simulink model "CAMFC2_04_simple_Formation"  (R2018b)
settings: Solver=ode23  StartTime=0.0  StopTime=20  RelTol=1e-3  EnableMultiTasking=on
InitFcn:
  | constant_CAMFC2_04_Simple_Formation
values from neighbouring files (symbols this model uses):
  alpha = 0.1    [constant_CAMFC2_01_WMR01.m]    (also in constant_CAMFC2_04_Comp.m = 0.01; constant_CAMFC2_04_Quad_03.m; constant_CAMFC2_04_Simple.m = 0.01; constant_CAMFC2_04_Simple_DoubleIntegrator.m = 0.01)
  AN = [     0 1 0 0 ... (first row only)    [constant_CAMFC2_01_WMR01.m]    (also in constant_CAMFC2_04_Comp.m = [     0 1 0 0 1; constant_CAMFC2_04_Quad_03.m; constant_CAMFC2_04_Simple.m; constant_CAMFC2_04_Simple_DoubleIntegrator.m)
  BN = [     1 0 0 0 ... (first row only)    [constant_CAMFC2_01_WMR01.m]    (also in constant_CAMFC2_04_Comp.m = [     0 0 0 0 0; constant_CAMFC2_04_Quad_03.m; constant_CAMFC2_04_Simple.m; constant_CAMFC2_04_Simple_DoubleIntegrator.m)
  chi = [0 0 0 0 ... (first row only)    [constant_CAMFC2_01_WMR01.m]    (also in constant_CAMFC2_04_Comp.m = X_m*ones(n0,1); constant_CAMFC2_04_Quad_03.m = X_m*ones(n0,1); constant_CAMFC2_04_Simple.m = X_m*ones(n0,1); constant_CAMFC2_04_Simple_DoubleIntegrator.m = X_m*ones(n0,1))
  epsilon_struct = struct('data',epsilon_InitVal)    [constant_CAMFC2_01_WMR01.m]    (also in constant_CAMFC2_04_Comp.m; constant_CAMFC2_04_Quad_03.m; constant_CAMFC2_04_Simple.m; constant_CAMFC2_04_Simple_DoubleIntegrator.m)
  gama1 = 1e4*diag([1e-6*ones(2,1);1e0*ones(2,1)])    [constant_CAMFC2_01_WMR01.m]    (also in constant_CAMFC2_04_Comp.m = 1e+3*diag([1e-6;1e-0]); constant_CAMFC2_04_Quad_03.m = 1e+2*diag(1e-0*ones(n0,1)); constant_CAMFC2_04_Simple.m = 1e+2*diag([1e-0;1e-0]); constant_CAMFC2_04_Simple_Formation.m = 1e+2*diag([1e-0;1e-0]))
  gama2 = 1e-2*diag([1e-6*ones(2,1);1e0*ones(2,1)])    [constant_CAMFC2_01_WMR01.m]    (also in constant_CAMFC2_04_Comp.m = 1e+0*diag([1e-6;1e-0]); constant_CAMFC2_04_Quad_03.m = 1e+0*diag(1e-0*ones(n0,1)); constant_CAMFC2_04_Simple.m = 1e+1*diag([1e-0;1e-0]); constant_CAMFC2_04_Simple_Formation.m = 1e+1*diag([1e-0;1e-0]))
  H = L + BN    [constant_CAMFC2_01_WMR01.m]    (also in constant_CAMFC2_04_Comp.m; constant_CAMFC2_04_Quad_03.m; constant_CAMFC2_04_Simple.m; constant_CAMFC2_04_Simple_DoubleIntegrator.m)
  k1 = 1    [constant_CAMFC2_01_WMR01.m]    (also in constant_CAMFC2_04_Comp.m; constant_CAMFC2_04_Quad_03.m = 50; constant_CAMFC2_04_Simple.m; constant_CAMFC2_04_Simple_DoubleIntegrator.m)
  k2 = 1    [constant_CAMFC2_01_WMR01.m]    (also in constant_CAMFC2_04_Comp.m; constant_CAMFC2_04_Quad_03.m; constant_CAMFC2_04_Simple.m; constant_CAMFC2_04_Simple_DoubleIntegrator.m)
  n = 4    [constant_CAMFC2_01_WMR01.m]    (also in constant_CAMFC2_04_Comp.m = 2; constant_CAMFC2_04_Quad_03.m = 6; constant_CAMFC2_04_Simple.m = 2; constant_CAMFC2_04_Simple_DoubleIntegrator.m = 2)
  N = 4    [constant_CAMFC2_01_WMR01.m]    (also in constant_CAMFC2_04_Comp.m = 5; constant_CAMFC2_04_Quad_03.m; constant_CAMFC2_04_Simple.m; constant_CAMFC2_04_Simple_DoubleIntegrator.m)
  n0 = 2    [constant_CAMFC2_01_WMR01.m]    (also in constant_CAMFC2_04_Comp.m = 1; constant_CAMFC2_04_Quad_03.m = 3; constant_CAMFC2_04_Simple.m; constant_CAMFC2_04_Simple_DoubleIntegrator.m = 1)
  Observer_Gain = 100    [constant_CAMFC2_01_WMR01.m]    (also in constant_CAMFC2_04_Comp.m = 10; constant_CAMFC2_04_Quad_03.m = 1; constant_CAMFC2_04_Simple.m; constant_CAMFC2_04_Simple_DoubleIntegrator.m)
  Observer_Gain1 = 100    [constant_CAMFC2_01_WMR01.m]    (also in constant_CAMFC2_04_Comp.m = 10; constant_CAMFC2_04_Quad_03.m = 1; constant_CAMFC2_04_Simple.m; constant_CAMFC2_04_Simple_DoubleIntegrator.m)
  Omega = [0 0 ... (first row only)    [constant_CAMFC2_04_Comp.m]    (also in constant_CAMFC2_04_Simple.m; constant_CAMFC2_04_Simple_DoubleIntegrator.m; constant_CAMFC2_04_Simple_DoubleIntegrator_02.m; constant_CAMFC2_04_Simple_Formation.m)
  P_struct = struct('data',P_InitVal)    [constant_CAMFC2_01_WMR01.m]    (also in constant_CAMFC2_04_Comp.m; constant_CAMFC2_04_Quad_03.m; constant_CAMFC2_04_Simple.m; constant_CAMFC2_04_Simple_DoubleIntegrator.m)
  Q = 1e-0*eye(n)    [constant_CAMFC2_01_WMR01.m]    (also in constant_CAMFC2_04_Comp.m = 1.0e+2*eye(n); constant_CAMFC2_04_Quad_03.m = 1e-0*eye(n0); constant_CAMFC2_04_Simple.m = 1.0e+1*eye(n); constant_CAMFC2_04_Simple_Formation.m = 1.0e+1*eye(n))
  rho1 = 1e-1    (= 0.1)    [constant_CAMFC2_01_WMR01.m]    (also in constant_CAMFC2_04_Comp.m = 1; constant_CAMFC2_04_Quad_03.m = 1; constant_CAMFC2_04_Simple.m = 1; constant_CAMFC2_04_Simple_DoubleIntegrator.m = 1)
  rho2 = 1e-3    (= 0.001)    [constant_CAMFC2_01_WMR01.m]    (also in constant_CAMFC2_04_Comp.m = 1; constant_CAMFC2_04_Quad_03.m = 1; constant_CAMFC2_04_Simple.m = 1; constant_CAMFC2_04_Simple_DoubleIntegrator.m = 10)
  T_struct = struct('data',T_InitVal)    [constant_CAMFC2_01_WMR01.m]    (also in constant_CAMFC2_04_Comp.m; constant_CAMFC2_04_Quad_03.m; constant_CAMFC2_04_Simple.m; constant_CAMFC2_04_Simple_DoubleIntegrator.m)
  Upsilon_M = Upsilon_m*ones(n,1)    [constant_CAMFC2_01_WMR01.m]    (also in constant_CAMFC2_04_Comp.m; constant_CAMFC2_04_Quad_03.m = Upsilon_m*ones(n0,1); constant_CAMFC2_04_Simple.m; constant_CAMFC2_04_Simple_DoubleIntegrator.m)
(part 1 of 3)
settings Model: ExtModeTrigDuration=100  Creator=hp  LastModifiedBy=ali
settings DataIOCC: LimitDataPoints=on  SaveFinalState=on  SaveFormat=StructureWithTime  SaveOutput=off  SaveState=on  StateSaveName=tmp_raccel_xout  SignalLoggingName=tmp_raccel_logsout
settings OptimizationCC: EfficientMapNaN2IntZero=off  LifeSpan=inf
settings DebuggingCC: UnderspecifiedInitializationDetection=Classic  MergeDetectMultiDrivingBlocksExec=none  SFUnexpectedBacktrackingDiag=warning  SFNoUnconditionalDefaultTransitionDiag=warning  SFExecutionAtInitializationDiag=none
settings HardwareCC: ProdBitPerPointer=32  ProdBitPerSizeT=32  ProdBitPerPtrDiffT=32  ProdLargestAtomicFloat=None  ProdIntDivRoundTo=Undefined  ProdEndianess=Unspecified  ProdWordSize=32  ProdHWDeviceType=32-bit Generic  TargetBitPerPointer=64  TargetBitPerSizeT=64  TargetBitPerPtrDiffT=64  TargetLongLongMode=on  TargetIntDivRoundTo=Zero  TargetEndianess=LittleEndian  TargetWordSize=64  TargetHWDeviceType=MATLAB Host  ProdEqTarget=off
settings ModelReferenceCC: PropagateSignalLabelsOutOfModel=off
settings SFSimCC: SimUseLocalCustomCode=off
settings RTWCC: SystemTargetFile=raccel.tlc  TemplateMakefile=raccel_default_tmf  RTWVerbose=off  RTWUseLocalCustomCode=off  RTWUseSimCustomCode=on
settings CodeAppCC: GenerateComments=off  MaxIdLength=128  MangleLength=10  SimulinkBlockComments=off
settings RaccelTargetCC: GeneratePreprocessorConditionals=Use local settings  MultiInstanceERTCode=off  PreserveStateflowLocalDataDimensions=off  ExtModeMexArgs='', 0, 54523  ENABLE_SLEXEC_SSBRIDGE=0  RTWCAPIParams=on
settings ConfigComp: CovMetricSettings=dw  CovHtmlReporting=on  CovSaveCumulativeToWorkspaceVar=on  CovSaveSingleToWorkspaceVar=on  CovExternalEMLEnable=off

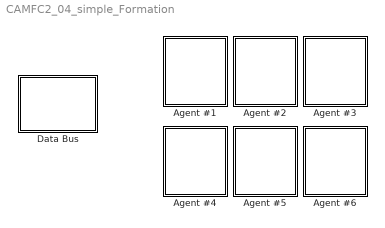
== system CAMFC2_04_simple_Formation ==
  Agent #1 : Subsystem
  Agent #2 : Subsystem
  Agent #3 : Subsystem
  Agent #4 : Subsystem
  Agent #5 : Subsystem
  Agent #6 : Subsystem
  "Data Bus " : Subsystem

== system CAMFC2_04_simple_Formation/Agent #1 ==
  Agent # : Constant
  Controller interpreter : MATLAB Function  TreatAsAtomicUnit=on
  Decenteralized Cooperaive Controller #1 : Subsystem
  Formation Plant : Subsystem
  tag scope: u1=global, x1=global
  wires:
  Decenteralized Cooperaive Controller #1/1(U1) -> Controller interpreter/1(U)
  Agent #/1 -> Decenteralized Cooperaive Controller #1/1(Agent #)
  Formation Plant/1(Y) -> [x1]
  Controller interpreter/1(u) -> Formation Plant/1(U), [u1]

== system CAMFC2_04_simple_Formation/Agent #2 ==
  Agent # : Constant  Value=2
  Controller interpreter : MATLAB Function  TreatAsAtomicUnit=on
  Decenteralized Cooperaive Controller #2 : Subsystem
  Formation Plant : Subsystem
  tag scope: u2=global, x2=global
  wires:
  Agent #/1 -> Decenteralized Cooperaive Controller #2/1(Agent #)
  Controller interpreter/1(u) -> Formation Plant/1(U), [u2]
  Formation Plant/1(Y) -> [x2]
  Decenteralized Cooperaive Controller #2/1(U2) -> Controller interpreter/1(U)

== system CAMFC2_04_simple_Formation/Agent #3 ==
  Agent # : Constant  Value=3
  Controller interpreter : MATLAB Function  TreatAsAtomicUnit=on
  Decenteralized Cooperaive Controller #3 : Subsystem
  Formation Plant : Subsystem
  tag scope: u3=global, x3=global
  wires:
  Agent #/1 -> Decenteralized Cooperaive Controller #3/1(Agent #)
  Formation Plant/1(Y) -> [x3]
  Decenteralized Cooperaive Controller #3/1(U3) -> Controller interpreter/1(U)
  Controller interpreter/1(u) -> Formation Plant/1(U), [u3]

== system CAMFC2_04_simple_Formation/Agent #4 ==
  Agent # : Constant  Value=4
  Controller interpreter : MATLAB Function  TreatAsAtomicUnit=on
  Decenteralized Cooperaive Controller #4 : Subsystem
  Formation Plant : Subsystem
  tag scope: u4=global, x4=global
  wires:
  Formation Plant/1(Y) -> [x4]
  Agent #/1 -> Decenteralized Cooperaive Controller #4/1(Agent #)
  Decenteralized Cooperaive Controller #4/1(U4) -> Controller interpreter/1(U)
  Controller interpreter/1(u) -> Formation Plant/1(U), [u4]

== system CAMFC2_04_simple_Formation/Agent #5 ==
  Agent # : Constant  Value=5
  Controller interpreter : MATLAB Function  TreatAsAtomicUnit=on
  Decenteralized Cooperaive Controller #5 : Subsystem
  Formation Plant : Subsystem
  tag scope: u5=global, x5=global
  wires:
  Controller interpreter/1(u) -> [u5], Formation Plant/1(U)
  Decenteralized Cooperaive Controller #5/1(U5) -> Controller interpreter/1(U)
  Agent #/1 -> Decenteralized Cooperaive Controller #5/1(Agent #)
  Formation Plant/1(Y) -> [x5]

== system CAMFC2_04_simple_Formation/Agent #6 ==
  Agent # : Constant  Value=6
  Controller interpreter : MATLAB Function  TreatAsAtomicUnit=on
  Decenteralized Cooperaive Controller #6 : Subsystem
  Formation Plant : Subsystem
  tag scope: u6=global, x6=global
  wires:
  Formation Plant/1(Y) -> [x6]
  Agent #/1 -> Decenteralized Cooperaive Controller #6/1(Agent #)
  Decenteralized Cooperaive Controller #6/1(U6) -> Controller interpreter/1(U)
  Controller interpreter/1(u) -> Formation Plant/1(U), [u6]

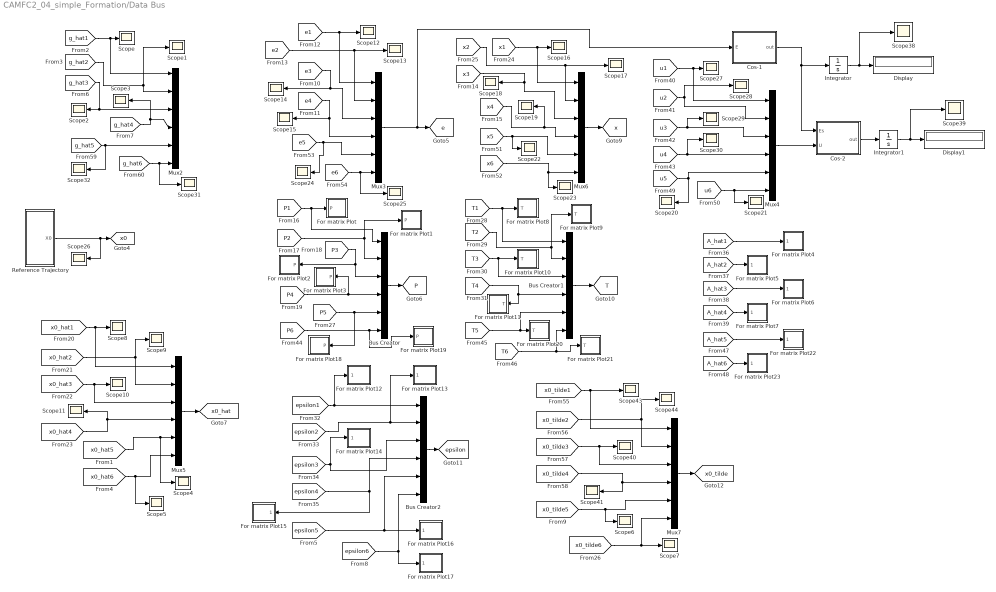
== system CAMFC2_04_simple_Formation/Data Bus  ==
  Bus Creator : BusCreator  Inputs=6  OutDataTypeStr=Bus: P_bus
  Bus Creator1 : BusCreator  Inputs=6  OutDataTypeStr=Bus: T_bus
  Bus Creator2 : BusCreator  Inputs=6  OutDataTypeStr=Bus: epsilon_bus
  Cos-1 : MATLAB Function  TreatAsAtomicUnit=on
  Cos-2 : MATLAB Function  TreatAsAtomicUnit=on
  Display : Display
  Display1 : Display
  For matrix Plot : Subsystem
  For matrix Plot1 : Subsystem
  For matrix Plot10 : Subsystem
  For matrix Plot11 : Subsystem
  For matrix Plot12 : Subsystem
  For matrix Plot13 : Subsystem
  For matrix Plot14 : Subsystem
  For matrix Plot15 : Subsystem
  For matrix Plot16 : Subsystem
  For matrix Plot17 : Subsystem
  For matrix Plot18 : Subsystem
  For matrix Plot19 : Subsystem
  For matrix Plot2 : Subsystem
  For matrix Plot20 : Subsystem
  For matrix Plot21 : Subsystem
  For matrix Plot22 : Subsystem
  For matrix Plot23 : Subsystem
  For matrix Plot3 : Subsystem
  For matrix Plot4 : Subsystem
  For matrix Plot5 : Subsystem
  For matrix Plot6 : Subsystem
  For matrix Plot7 : Subsystem
  For matrix Plot8 : Subsystem
  For matrix Plot9 : Subsystem
  Integrator : Integrator
  Integrator1 : Integrator
  Mux{2..7} (6 alike) : Mux  Inputs=6
  Reference Trajectory : Subsystem
  Scope{,1..32,38..41,43..44} (39 alike) : Scope
  tag scope: P=global, T=global, e=global, epsilon=global, x0=global, x0_hat=global, x0_tilde=global, x=global
  wires:
  [g_hat2] -> Scope1/1, Mux2/2
  [g_hat1] -> Mux2/1, Scope/1
  [e2] -> Mux3/2, Scope13/1
  [e1] -> Mux3/1, Scope12/1
  Mux3/1 -> Cos-1/1(E), [e]
  [P2] -> Bus Creator/2, For matrix Plot1/1(P)
  [P1] -> Bus Creator/1, For matrix Plot/1(P)
  Bus Creator/1 -> [P]
  [x0_hat2] -> Scope9/1, Mux5/2
  [x0_hat1] -> Mux5/1, Scope8/1
  Mux5/1 -> [x0_hat]
  Reference Trajectory/1(X0) -> [x0], Scope26/1
  [x2] -> Mux6/2, Scope17/1
  [x1] -> Mux6/1, Scope16/1
  Mux6/1 -> [x]
  [g_hat3] -> Mux2/3, Scope2/1
  [g_hat4] -> Mux2/4, Scope3/1
  [e3] -> Mux3/3, Scope14/1
  [e4] -> Mux3/4, Scope15/1
  [x3] -> Mux6/3, Scope18/1
  [x4] -> Mux6/4, Scope19/1
  [P3] -> Bus Creator/3, For matrix Plot2/1(P)
  [P4] -> For matrix Plot3/1(P), Bus Creator/4
  [x0_hat3] -> Mux5/3, Scope10/1
  [x0_hat4] -> Scope11/1, Mux5/4
  [T2] -> Bus Creator1/2, For matrix Plot9/1(T)
  [T1] -> Bus Creator1/1, For matrix Plot8/1(T)
  Bus Creator1/1 -> [T]
  [T3] -> Bus Creator1/3, For matrix Plot10/1(T)
  [T4] -> For matrix Plot11/1(T), Bus Creator1/4
  [epsilon2] -> Bus Creator2/2, For matrix Plot13/1(epsilon)
  [epsilon1] -> Bus Creator2/1, For matrix Plot12/1(epsilon)
  Bus Creator2/1 -> [epsilon]
  [epsilon3] -> For matrix Plot14/1(epsilon), Bus Creator2/3
  [epsilon4] -> For matrix Plot15/1(epsilon), Bus Creator2/4
  [A_hat2] -> For matrix Plot5/1(A_hat)
  [A_hat1] -> For matrix Plot4/1(A_hat)
  [A_hat3] -> For matrix Plot6/1(A_hat)
  [A_hat4] -> For matrix Plot7/1(A_hat)
  [u2] -> Mux4/2, Scope28/1
  [u1] -> Mux4/1, Scope27/1
  [u4] -> Mux4/4, Scope30/1
  Integrator/1 -> Scope38/1, Display/1
  Cos-1/1(out) -> Integrator/1, Cos-2/1(Es)
  [u3] -> Mux4/3, Scope29/1
  Mux4/1 -> Cos-2/2(U)
  Integrator1/1 -> Display1/1, Scope39/1
  Cos-2/1(out) -> Integrator1/1
  [x0_tilde4] -> Scope41/1, Mux7/4
  [x0_tilde1] -> Mux7/1, Scope43/1
  [x0_tilde3] -> Mux7/3, Scope40/1
  [x0_tilde2] -> Mux7/2, Scope44/1
  Mux7/1 -> [x0_tilde]
  [x0_hat5] -> Scope4/1, Mux5/5
  [x0_hat6] -> Scope5/1, Mux5/6
  [epsilon5] -> For matrix Plot16/1(epsilon), Bus Creator2/5
  [epsilon6] -> For matrix Plot17/1(epsilon), Bus Creator2/6
  [x0_tilde5] -> Scope6/1, Mux7/5
  [x0_tilde6] -> Scope7/1, Mux7/6
  [P5] -> Bus Creator/5, For matrix Plot18/1(P)
  [P6] -> For matrix Plot19/1(P), Bus Creator/6
  [T5] -> For matrix Plot20/1(T), Bus Creator1/5
  [T6] -> For matrix Plot21/1(T), Bus Creator1/6
  [A_hat5] -> For matrix Plot22/1(A_hat)
  [A_hat6] -> For matrix Plot23/1(A_hat)
  [u5] -> Scope20/1, Mux4/5
  [u6] -> Scope21/1, Mux4/6
  [x5] -> Scope22/1, Mux6/5
  [x6] -> Scope23/1, Mux6/6
  [e5] -> Scope24/1, Mux3/5
  [e6] -> Scope25/1, Mux3/6
  [g_hat5] -> Scope32/1, Mux2/5
  [g_hat6] -> Scope31/1, Mux2/6

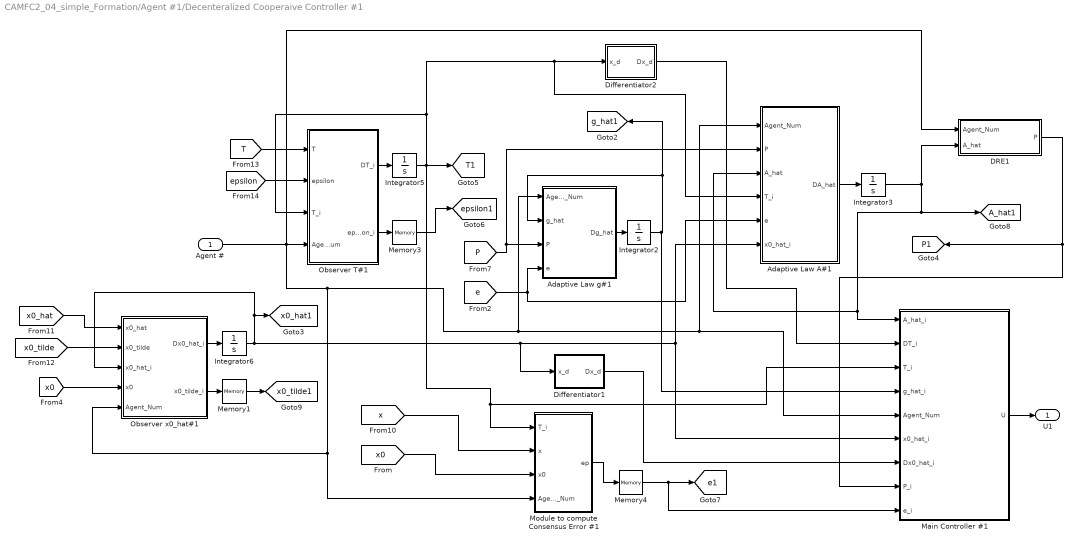
== system CAMFC2_04_simple_Formation/Agent #1/Decenteralized Cooperaive Controller #1 ==
  Agent # : Inport
  Adaptive Law A#1 : MATLAB Function  TreatAsAtomicUnit=on
  Adaptive Law g#1 : MATLAB Function  TreatAsAtomicUnit=on
  DRE1 : Subsystem
  Differentiator1 : Subsystem
  Differentiator2 : Subsystem
  Integrator2 : Integrator  InitialCondition=zeros(n,1)
  Integrator3 : Integrator  InitialCondition=zeros(n)
  Integrator5 : Integrator  InitialCondition=zeros(N+1,n)
  Integrator6 : Integrator  InitialCondition=zeros(n0,1)
  Main Controller #1 : MATLAB Function  TreatAsAtomicUnit=on
  Memory1 : Memory  InitialCondition=zeros(n0,1)
  Memory3 : Memory  InitialCondition=zeros(N+1,n)
  Memory4 : Memory  InitialCondition=zeros(n,1)
  Module to compute Consensus Error #1 : MATLAB Function  TreatAsAtomicUnit=on
  Observer T#1 : MATLAB Function  TreatAsAtomicUnit=on
  Observer x0_hat#1 : MATLAB Function  TreatAsAtomicUnit=on
  U1 : Outport
  tag scope: A_hat1=global, P1=global, T1=global, e1=global, epsilon1=global, g_hat1=global, x0_hat1=global, x0_tilde1=global
  wires:
  [x] -> Module to compute Consensus Error #1/2(x)
  Module to compute Consensus Error #1/1(ep) -> Memory4/1
  [x0] -> Module to compute Consensus Error #1/3(x0)
  Differentiator2/1(Dx_d) -> Main Controller #1/2(DT_i)
  [epsilon] -> Observer T#1/2(epsilon)
  [T] -> Observer T#1/1(T)
  Memory3/1 -> [epsilon1]
  Observer T#1/2(epsilon_i) -> Memory3/1
  Integrator5/1 -> Module to compute Consensus Error #1/1(T_i), Main Controller #1/3(T_i), [T1], Adaptive Law A#1/4(T_i), Differentiator2/1(x_d), Observer T#1/3(T_i)
  Observer T#1/1(DT_i) -> Integrator5/1
  Memory4/1 -> [e1], Main Controller #1/9(e_i)
  Integrator3/1 -> DRE1/2(A_hat), Adaptive Law A#1/3(A_hat), Main Controller #1/1(A_hat_i), [A_hat1]
  [e] -> Adaptive Law A#1/5(e), Adaptive Law g#1/4(e)
  [P] -> Adaptive Law A#1/2(P), Adaptive Law g#1/3(P)
  DRE1/1(P) -> [P1], Main Controller #1/8(P_i)
  Integrator2/1 -> Main Controller #1/4(g_hat_i), Adaptive Law g#1/2(g_hat), [g_hat1]
  Adaptive Law g#1/1(Dg_hat) -> Integrator2/1
  Main Controller #1/1(U) -> U1/1
  Adaptive Law A#1/1(DA_hat) -> Integrator3/1
  Agent #/1 -> DRE1/1(Agent_Num), Observer T#1/4(Agent_Num), Observer x0_hat#1/5(Agent_Num), Module to compute Consensus Error #1/4(Agent_Num), Adaptive Law g#1/1(Agent_Num), Main Controller #1/5(Agent_Num), Adaptive Law A#1/1(Agent_Num)
  Observer x0_hat#1/2(x0_tilde_i) -> Memory1/1
  Memory1/1 -> [x0_tilde1]
  Observer x0_hat#1/1(Dx0_hat_i) -> Integrator6/1
  [x0_tilde] -> Observer x0_hat#1/2(x0_tilde)
  [x0] -> Observer x0_hat#1/4(x0)
  [x0_hat] -> Observer x0_hat#1/1(x0_hat)
  Integrator6/1 -> Observer x0_hat#1/3(x0_hat_i), [x0_hat1], Differentiator1/1(x_d), Main Controller #1/6(x0_hat_i), Adaptive Law A#1/6(x0_hat_i)
  Differentiator1/1(Dx_d) -> Main Controller #1/7(Dx0_hat_i)

== system CAMFC2_04_simple_Formation/Agent #1/Formation Plant ==
  U : Inport
  Plant : Subsystem
  Y : Outport
  wires:
  U/1 -> Plant/1(U)
  Plant/1(Y) -> Y/1

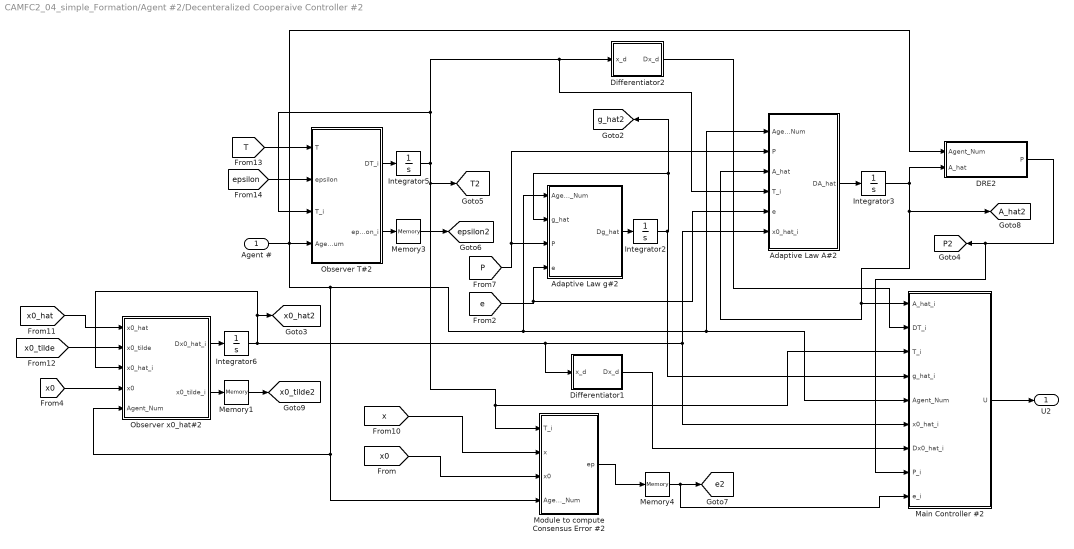
== system CAMFC2_04_simple_Formation/Agent #2/Decenteralized Cooperaive Controller #2 ==
  Agent # : Inport
  Adaptive Law A#2 : MATLAB Function  TreatAsAtomicUnit=on
  Adaptive Law g#2 : MATLAB Function  TreatAsAtomicUnit=on
  DRE2 : Subsystem
  Differentiator1 : Subsystem
  Differentiator2 : Subsystem
  Integrator2 : Integrator  InitialCondition=zeros(n,1)
  Integrator3 : Integrator  InitialCondition=zeros(n)
  Integrator5 : Integrator  InitialCondition=zeros(N+1,n)
  Integrator6 : Integrator  InitialCondition=zeros(n0,1)
  Main Controller #2 : MATLAB Function  TreatAsAtomicUnit=on
  Memory1 : Memory  InitialCondition=zeros(n0,1)
  Memory3 : Memory  InitialCondition=zeros(N+1,n)
  Memory4 : Memory  InitialCondition=zeros(n,1)
  Module to compute Consensus Error #2 : MATLAB Function  TreatAsAtomicUnit=on
  Observer T#2 : MATLAB Function  TreatAsAtomicUnit=on
  Observer x0_hat#2 : MATLAB Function  TreatAsAtomicUnit=on
  U2 : Outport
  tag scope: A_hat2=global, P2=global, T2=global, e2=global, epsilon2=global, g_hat2=global, x0_hat2=global, x0_tilde2=global
  wires:
  [x] -> Module to compute Consensus Error #2/2(x)
  Module to compute Consensus Error #2/1(ep) -> Memory4/1
  [x0] -> Module to compute Consensus Error #2/3(x0)
  Differentiator2/1(Dx_d) -> Main Controller #2/2(DT_i)
  [epsilon] -> Observer T#2/2(epsilon)
  [T] -> Observer T#2/1(T)
  Memory3/1 -> [epsilon2]
  Observer T#2/2(epsilon_i) -> Memory3/1
  Integrator5/1 -> [T2], Main Controller #2/3(T_i), Module to compute Consensus Error #2/1(T_i), Adaptive Law A#2/4(T_i), Differentiator2/1(x_d), Observer T#2/3(T_i)
  Observer T#2/1(DT_i) -> Integrator5/1
  Memory4/1 -> Main Controller #2/9(e_i), [e2]
  Integrator3/1 -> DRE2/2(A_hat), [A_hat2], Main Controller #2/1(A_hat_i), Adaptive Law A#2/3(A_hat)
  [e] -> Adaptive Law A#2/5(e), Adaptive Law g#2/4(e)
  [P] -> Adaptive Law A#2/2(P), Adaptive Law g#2/3(P)
  DRE2/1(P) -> Main Controller #2/8(P_i), [P2]
  Integrator2/1 -> Main Controller #2/4(g_hat_i), Adaptive Law g#2/2(g_hat), [g_hat2]
  Adaptive Law g#2/1(Dg_hat) -> Integrator2/1
  Main Controller #2/1(U) -> U2/1
  Adaptive Law A#2/1(DA_hat) -> Integrator3/1
  Agent #/1 -> DRE2/1(Agent_Num), Observer T#2/4(Agent_Num), Observer x0_hat#2/5(Agent_Num), Module to compute Consensus Error #2/4(Agent_Num), Adaptive Law g#2/1(Agent_Num), Main Controller #2/5(Agent_Num), Adaptive Law A#2/1(Agent_Num)
  Observer x0_hat#2/2(x0_tilde_i) -> Memory1/1
  Memory1/1 -> [x0_tilde2]
  Observer x0_hat#2/1(Dx0_hat_i) -> Integrator6/1
  [x0_tilde] -> Observer x0_hat#2/2(x0_tilde)
  [x0] -> Observer x0_hat#2/4(x0)
  [x0_hat] -> Observer x0_hat#2/1(x0_hat)
  Integrator6/1 -> Observer x0_hat#2/3(x0_hat_i), [x0_hat2], Differentiator1/1(x_d), Main Controller #2/6(x0_hat_i), Adaptive Law A#2/6(x0_hat_i)
  Differentiator1/1(Dx_d) -> Main Controller #2/7(Dx0_hat_i)

== system CAMFC2_04_simple_Formation/Agent #2/Formation Plant ==
  U : Inport
  Plant : Subsystem
  Y : Outport
  wires:
  U/1 -> Plant/1(U)
  Plant/1(Y) -> Y/1

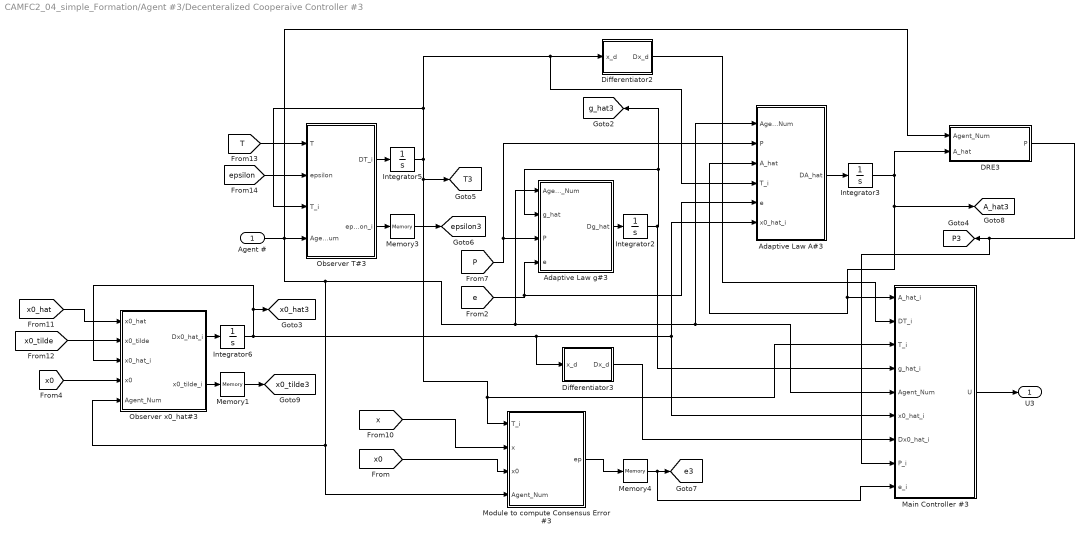
== system CAMFC2_04_simple_Formation/Agent #3/Decenteralized Cooperaive Controller #3 ==
  Agent # : Inport
  Adaptive Law A#3 : MATLAB Function  TreatAsAtomicUnit=on
  Adaptive Law g#3 : MATLAB Function  TreatAsAtomicUnit=on
  DRE3 : Subsystem
  Differentiator2 : Subsystem
  Differentiator3 : Subsystem
  Integrator2 : Integrator  InitialCondition=zeros(n,1)
  Integrator3 : Integrator  InitialCondition=zeros(n)
  Integrator5 : Integrator  InitialCondition=zeros(N+1,n)
  Integrator6 : Integrator  InitialCondition=zeros(n0,1)
  Main Controller #3 : MATLAB Function  TreatAsAtomicUnit=on
  Memory1 : Memory  InitialCondition=zeros(n0,1)
  Memory3 : Memory  InitialCondition=zeros(N+1,n)
  Memory4 : Memory  InitialCondition=zeros(n,1)
  Module to compute Consensus Error #3 : MATLAB Function  TreatAsAtomicUnit=on
  Observer T#3 : MATLAB Function  TreatAsAtomicUnit=on
  Observer x0_hat#3 : MATLAB Function  TreatAsAtomicUnit=on
  U3 : Outport
  tag scope: A_hat3=global, P3=global, T3=global, e3=global, epsilon3=global, g_hat3=global, x0_hat3=global, x0_tilde3=global
  wires:
  [x] -> Module to compute Consensus Error #3/2(x)
  Module to compute Consensus Error #3/1(ep) -> Memory4/1
  [x0] -> Module to compute Consensus Error #3/3(x0)
  Differentiator2/1(Dx_d) -> Main Controller #3/2(DT_i)
  [epsilon] -> Observer T#3/2(epsilon)
  [T] -> Observer T#3/1(T)
  Memory3/1 -> [epsilon3]
  Observer T#3/2(epsilon_i) -> Memory3/1
  Integrator5/1 -> [T3], Main Controller #3/3(T_i), Module to compute Consensus Error #3/1(T_i), Adaptive Law A#3/4(T_i), Differentiator2/1(x_d), Observer T#3/3(T_i)
  Observer T#3/1(DT_i) -> Integrator5/1
  Memory4/1 -> Main Controller #3/9(e_i), [e3]
  Integrator3/1 -> DRE3/2(A_hat), [A_hat3], Main Controller #3/1(A_hat_i), Adaptive Law A#3/3(A_hat)
  [e] -> Adaptive Law A#3/5(e), Adaptive Law g#3/4(e)
  [P] -> Adaptive Law A#3/2(P), Adaptive Law g#3/3(P)
  DRE3/1(P) -> Main Controller #3/8(P_i), [P3]
  Integrator2/1 -> Main Controller #3/4(g_hat_i), Adaptive Law g#3/2(g_hat), [g_hat3]
  Adaptive Law g#3/1(Dg_hat) -> Integrator2/1
  Main Controller #3/1(U) -> U3/1
  Adaptive Law A#3/1(DA_hat) -> Integrator3/1
  Agent #/1 -> DRE3/1(Agent_Num), Observer T#3/4(Agent_Num), Observer x0_hat#3/5(Agent_Num), Module to compute Consensus Error #3/4(Agent_Num), Adaptive Law g#3/1(Agent_Num), Main Controller #3/5(Agent_Num), Adaptive Law A#3/1(Agent_Num)
  Observer x0_hat#3/2(x0_tilde_i) -> Memory1/1
  Memory1/1 -> [x0_tilde3]
  Observer x0_hat#3/1(Dx0_hat_i) -> Integrator6/1
  [x0_tilde] -> Observer x0_hat#3/2(x0_tilde)
  [x0] -> Observer x0_hat#3/4(x0)
  [x0_hat] -> Observer x0_hat#3/1(x0_hat)
  Integrator6/1 -> Observer x0_hat#3/3(x0_hat_i), [x0_hat3], Differentiator3/1(x_d), Main Controller #3/6(x0_hat_i), Adaptive Law A#3/6(x0_hat_i)
  Differentiator3/1(Dx_d) -> Main Controller #3/7(Dx0_hat_i)

== system CAMFC2_04_simple_Formation/Agent #3/Formation Plant ==
  U : Inport
  Plant : Subsystem
  Y : Outport
  wires:
  U/1 -> Plant/1(U)
  Plant/1(Y) -> Y/1

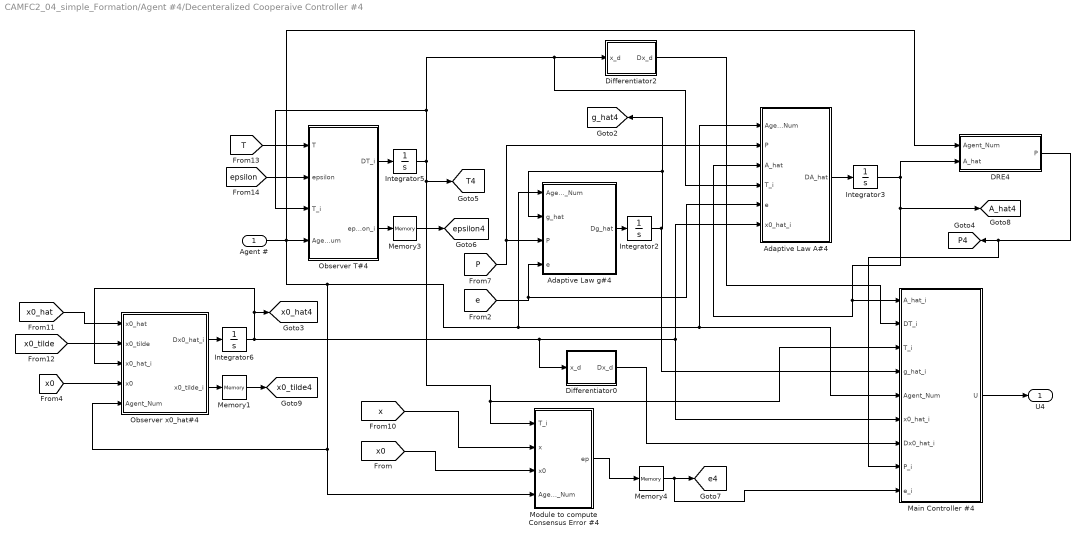
== system CAMFC2_04_simple_Formation/Agent #4/Decenteralized Cooperaive Controller #4 ==
  Agent # : Inport
  Adaptive Law A#4 : MATLAB Function  TreatAsAtomicUnit=on
  Adaptive Law g#4 : MATLAB Function  TreatAsAtomicUnit=on
  DRE4 : Subsystem
  Differentiator0 : Subsystem
  Differentiator2 : Subsystem
  Integrator2 : Integrator  InitialCondition=zeros(n,1)
  Integrator3 : Integrator  InitialCondition=zeros(n)
  Integrator5 : Integrator  InitialCondition=zeros(N+1,n)
  Integrator6 : Integrator  InitialCondition=zeros(n0,1)
  Main Controller #4 : MATLAB Function  TreatAsAtomicUnit=on
  Memory1 : Memory  InitialCondition=zeros(n0,1)
  Memory3 : Memory  InitialCondition=zeros(N+1,n)
  Memory4 : Memory  InitialCondition=zeros(n,1)
  Module to compute Consensus Error #4 : MATLAB Function  TreatAsAtomicUnit=on
  Observer T#4 : MATLAB Function  TreatAsAtomicUnit=on
  Observer x0_hat#4 : MATLAB Function  TreatAsAtomicUnit=on
  U4 : Outport
  tag scope: A_hat4=global, P4=global, T4=global, e4=global, epsilon4=global, g_hat4=global, x0_hat4=global, x0_tilde4=global
  wires:
  [x] -> Module to compute Consensus Error #4/2(x)
  Module to compute Consensus Error #4/1(ep) -> Memory4/1
  [x0] -> Module to compute Consensus Error #4/3(x0)
  Differentiator2/1(Dx_d) -> Main Controller #4/2(DT_i)
  [epsilon] -> Observer T#4/2(epsilon)
  [T] -> Observer T#4/1(T)
  Memory3/1 -> [epsilon4]
  Observer T#4/2(epsilon_i) -> Memory3/1
  Integrator5/1 -> [T4], Main Controller #4/3(T_i), Module to compute Consensus Error #4/1(T_i), Adaptive Law A#4/4(T_i), Differentiator2/1(x_d), Observer T#4/3(T_i)
  Observer T#4/1(DT_i) -> Integrator5/1
  Memory4/1 -> Main Controller #4/9(e_i), [e4]
  Integrator3/1 -> DRE4/2(A_hat), [A_hat4], Main Controller #4/1(A_hat_i), Adaptive Law A#4/3(A_hat)
  [e] -> Adaptive Law A#4/5(e), Adaptive Law g#4/4(e)
  [P] -> Adaptive Law A#4/2(P), Adaptive Law g#4/3(P)
  DRE4/1(P) -> Main Controller #4/8(P_i), [P4]
  Integrator2/1 -> Main Controller #4/4(g_hat_i), Adaptive Law g#4/2(g_hat), [g_hat4]
  Adaptive Law g#4/1(Dg_hat) -> Integrator2/1
  Main Controller #4/1(U) -> U4/1
  Adaptive Law A#4/1(DA_hat) -> Integrator3/1
  Agent #/1 -> DRE4/1(Agent_Num), Observer T#4/4(Agent_Num), Observer x0_hat#4/5(Agent_Num), Module to compute Consensus Error #4/4(Agent_Num), Adaptive Law g#4/1(Agent_Num), Main Controller #4/5(Agent_Num), Adaptive Law A#4/1(Agent_Num)
  Observer x0_hat#4/2(x0_tilde_i) -> Memory1/1
  Memory1/1 -> [x0_tilde4]
  Observer x0_hat#4/1(Dx0_hat_i) -> Integrator6/1
  [x0_tilde] -> Observer x0_hat#4/2(x0_tilde)
  [x0] -> Observer x0_hat#4/4(x0)
  [x0_hat] -> Observer x0_hat#4/1(x0_hat)
  Integrator6/1 -> Observer x0_hat#4/3(x0_hat_i), [x0_hat4], Differentiator0/1(x_d), Main Controller #4/6(x0_hat_i), Adaptive Law A#4/6(x0_hat_i)
  Differentiator0/1(Dx_d) -> Main Controller #4/7(Dx0_hat_i)

== system CAMFC2_04_simple_Formation/Agent #4/Formation Plant ==
  U : Inport
  Plant : Subsystem
  Y : Outport
  wires:
  U/1 -> Plant/1(U)
  Plant/1(Y) -> Y/1

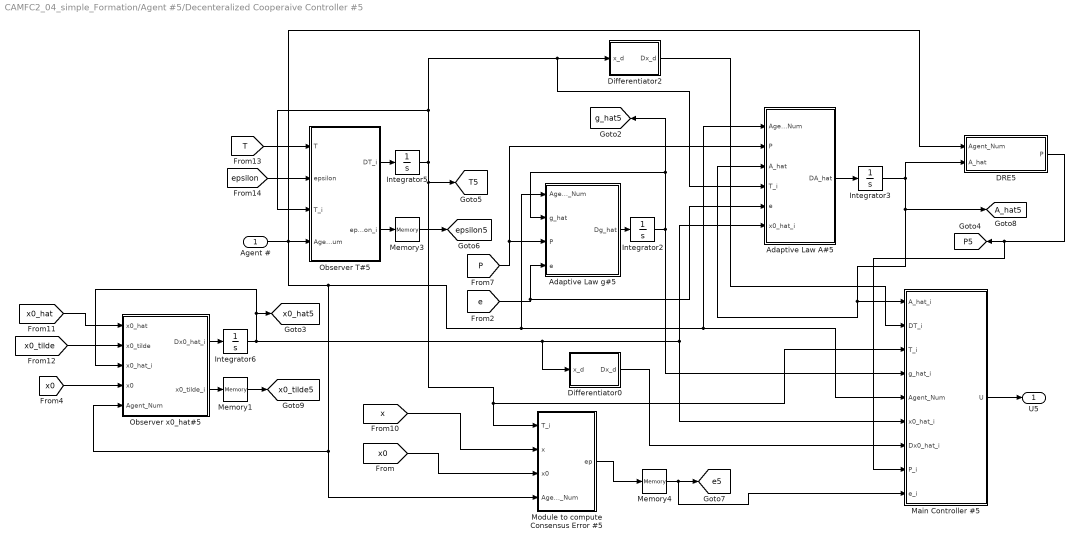
== system CAMFC2_04_simple_Formation/Agent #5/Decenteralized Cooperaive Controller #5 ==
  Agent # : Inport
  Adaptive Law A#5 : MATLAB Function  TreatAsAtomicUnit=on
  Adaptive Law g#5 : MATLAB Function  TreatAsAtomicUnit=on
  DRE5 : Subsystem
  Differentiator0 : Subsystem
  Differentiator2 : Subsystem
  Integrator2 : Integrator  InitialCondition=zeros(n,1)
  Integrator3 : Integrator  InitialCondition=zeros(n)
  Integrator5 : Integrator  InitialCondition=zeros(N+1,n)
  Integrator6 : Integrator  InitialCondition=zeros(n0,1)
  Main Controller #5 : MATLAB Function  TreatAsAtomicUnit=on
  Memory1 : Memory  InitialCondition=zeros(n0,1)
  Memory3 : Memory  InitialCondition=zeros(N+1,n)
  Memory4 : Memory  InitialCondition=zeros(n,1)
  Module to compute Consensus Error #5 : MATLAB Function  TreatAsAtomicUnit=on
  Observer T#5 : MATLAB Function  TreatAsAtomicUnit=on
  Observer x0_hat#5 : MATLAB Function  TreatAsAtomicUnit=on
  U5 : Outport
  tag scope: A_hat5=global, P5=global, T5=global, e5=global, epsilon5=global, g_hat5=global, x0_hat5=global, x0_tilde5=global
  wires:
  Differentiator0/1(Dx_d) -> Main Controller #5/7(Dx0_hat_i)
  Integrator6/1 -> Adaptive Law A#5/6(x0_hat_i), Main Controller #5/6(x0_hat_i), Differentiator0/1(x_d), [x0_hat5], Observer x0_hat#5/3(x0_hat_i)
  [x0_hat] -> Observer x0_hat#5/1(x0_hat)
  [x0] -> Observer x0_hat#5/4(x0)
  [x0_tilde] -> Observer x0_hat#5/2(x0_tilde)
  Observer x0_hat#5/1(Dx0_hat_i) -> Integrator6/1
  Memory1/1 -> [x0_tilde5]
  Observer x0_hat#5/2(x0_tilde_i) -> Memory1/1
  Agent #/1 -> Adaptive Law A#5/1(Agent_Num), Main Controller #5/5(Agent_Num), Adaptive Law g#5/1(Agent_Num), Module to compute Consensus Error #5/4(Agent_Num), Observer x0_hat#5/5(Agent_Num), Observer T#5/4(Agent_Num), DRE5/1(Agent_Num)
  Adaptive Law A#5/1(DA_hat) -> Integrator3/1
  Main Controller #5/1(U) -> U5/1
  Adaptive Law g#5/1(Dg_hat) -> Integrator2/1
  Integrator2/1 -> [g_hat5], Adaptive Law g#5/2(g_hat), Main Controller #5/4(g_hat_i)
  DRE5/1(P) -> [P5], Main Controller #5/8(P_i)
  [P] -> Adaptive Law g#5/3(P), Adaptive Law A#5/2(P)
  [e] -> Adaptive Law g#5/4(e), Adaptive Law A#5/5(e)
  Integrator3/1 -> Adaptive Law A#5/3(A_hat), Main Controller #5/1(A_hat_i), [A_hat5], DRE5/2(A_hat)
  Memory4/1 -> [e5], Main Controller #5/9(e_i)
  Observer T#5/1(DT_i) -> Integrator5/1
  Integrator5/1 -> Observer T#5/3(T_i), Differentiator2/1(x_d), Adaptive Law A#5/4(T_i), Module to compute Consensus Error #5/1(T_i), Main Controller #5/3(T_i), [T5]
  Observer T#5/2(epsilon_i) -> Memory3/1
  Memory3/1 -> [epsilon5]
  [T] -> Observer T#5/1(T)
  [epsilon] -> Observer T#5/2(epsilon)
  Differentiator2/1(Dx_d) -> Main Controller #5/2(DT_i)
  [x0] -> Module to compute Consensus Error #5/3(x0)
  Module to compute Consensus Error #5/1(ep) -> Memory4/1
  [x] -> Module to compute Consensus Error #5/2(x)

== system CAMFC2_04_simple_Formation/Agent #5/Formation Plant ==
  U : Inport
  Plant : Subsystem
  Y : Outport
  wires:
  Plant/1(Y) -> Y/1
  U/1 -> Plant/1(U)

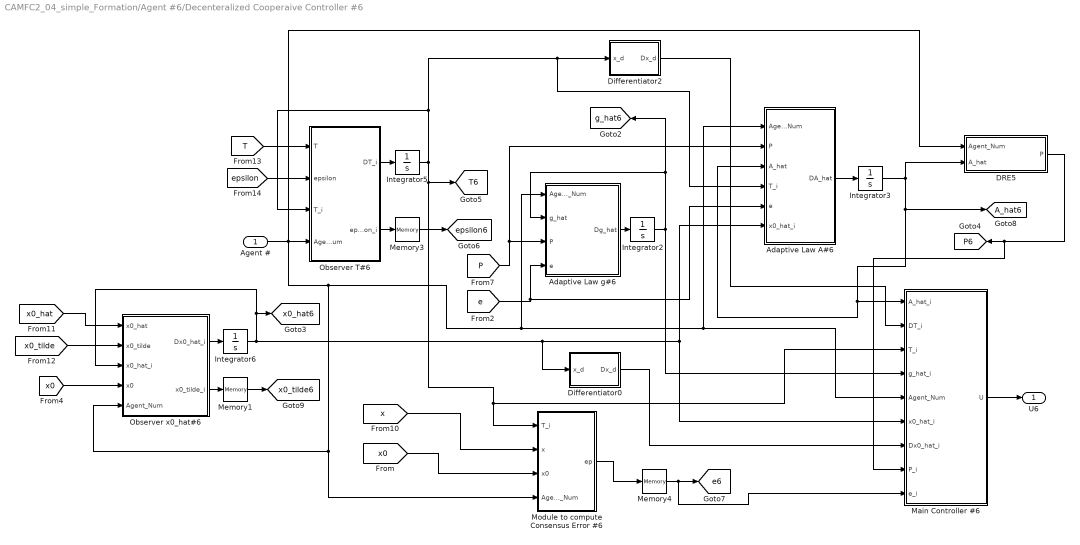
== system CAMFC2_04_simple_Formation/Agent #6/Decenteralized Cooperaive Controller #6 ==
  Agent # : Inport
  Adaptive Law A#6 : MATLAB Function  TreatAsAtomicUnit=on
  Adaptive Law g#6 : MATLAB Function  TreatAsAtomicUnit=on
  DRE5 : Subsystem
  Differentiator0 : Subsystem
  Differentiator2 : Subsystem
  Integrator2 : Integrator  InitialCondition=zeros(n,1)
  Integrator3 : Integrator  InitialCondition=zeros(n)
  Integrator5 : Integrator  InitialCondition=zeros(N+1,n)
  Integrator6 : Integrator  InitialCondition=zeros(n0,1)
  Main Controller #6 : MATLAB Function  TreatAsAtomicUnit=on
  Memory1 : Memory  InitialCondition=zeros(n0,1)
  Memory3 : Memory  InitialCondition=zeros(N+1,n)
  Memory4 : Memory  InitialCondition=zeros(n,1)
  Module to compute Consensus Error #6 : MATLAB Function  TreatAsAtomicUnit=on
  Observer T#6 : MATLAB Function  TreatAsAtomicUnit=on
  Observer x0_hat#6 : MATLAB Function  TreatAsAtomicUnit=on
  U6 : Outport
  tag scope: A_hat6=global, P6=global, T6=global, e6=global, epsilon6=global, g_hat6=global, x0_hat6=global, x0_tilde6=global
  wires:
  [x] -> Module to compute Consensus Error #6/2(x)
  Module to compute Consensus Error #6/1(ep) -> Memory4/1
  [x0] -> Module to compute Consensus Error #6/3(x0)
  Differentiator2/1(Dx_d) -> Main Controller #6/2(DT_i)
  [epsilon] -> Observer T#6/2(epsilon)
  [T] -> Observer T#6/1(T)
  Memory3/1 -> [epsilon6]
  Observer T#6/2(epsilon_i) -> Memory3/1
  Integrator5/1 -> [T6], Main Controller #6/3(T_i), Module to compute Consensus Error #6/1(T_i), Adaptive Law A#6/4(T_i), Differentiator2/1(x_d), Observer T#6/3(T_i)
  Observer T#6/1(DT_i) -> Integrator5/1
  Memory4/1 -> Main Controller #6/9(e_i), [e6]
  Integrator3/1 -> DRE5/2(A_hat), [A_hat6], Main Controller #6/1(A_hat_i), Adaptive Law A#6/3(A_hat)
  [e] -> Adaptive Law A#6/5(e), Adaptive Law g#6/4(e)
  [P] -> Adaptive Law A#6/2(P), Adaptive Law g#6/3(P)
  DRE5/1(P) -> Main Controller #6/8(P_i), [P6]
  Integrator2/1 -> Main Controller #6/4(g_hat_i), Adaptive Law g#6/2(g_hat), [g_hat6]
  Adaptive Law g#6/1(Dg_hat) -> Integrator2/1
  Main Controller #6/1(U) -> U6/1
  Adaptive Law A#6/1(DA_hat) -> Integrator3/1
  Agent #/1 -> DRE5/1(Agent_Num), Observer T#6/4(Agent_Num), Observer x0_hat#6/5(Agent_Num), Module to compute Consensus Error #6/4(Agent_Num), Adaptive Law g#6/1(Agent_Num), Main Controller #6/5(Agent_Num), Adaptive Law A#6/1(Agent_Num)
  Observer x0_hat#6/2(x0_tilde_i) -> Memory1/1
  Memory1/1 -> [x0_tilde6]
  Observer x0_hat#6/1(Dx0_hat_i) -> Integrator6/1
  [x0_tilde] -> Observer x0_hat#6/2(x0_tilde)
  [x0] -> Observer x0_hat#6/4(x0)
  [x0_hat] -> Observer x0_hat#6/1(x0_hat)
  Integrator6/1 -> Observer x0_hat#6/3(x0_hat_i), [x0_hat6], Differentiator0/1(x_d), Main Controller #6/6(x0_hat_i), Adaptive Law A#6/6(x0_hat_i)
  Differentiator0/1(Dx_d) -> Main Controller #6/7(Dx0_hat_i)

== system CAMFC2_04_simple_Formation/Agent #6/Formation Plant ==
  U : Inport
  Plant : Subsystem
  Y : Outport
  wires:
  U/1 -> Plant/1(U)
  Plant/1(Y) -> Y/1

== system CAMFC2_04_simple_Formation/Data Bus /For matrix Plot ==
  P : Inport
  MATLAB Function : MATLAB Function  TreatAsAtomicUnit=on
  Scope17 : Scope
  To Workspace : ToWorkspace  VariableName=P1  SaveFormat=Structure With Time  SampleTime=-1
  wires:
  P/1 -> MATLAB Function/1(u)
  MATLAB Function/1(y) -> Scope17/1, To Workspace/1

== system CAMFC2_04_simple_Formation/Data Bus /For matrix Plot1 ==
  P : Inport
  MATLAB Function : MATLAB Function  TreatAsAtomicUnit=on
  To Workspace : ToWorkspace  VariableName=P2  SaveFormat=Structure With Time  SampleTime=-1
  wires:
  MATLAB Function/1(y) -> To Workspace/1
  P/1 -> MATLAB Function/1(u)

== system CAMFC2_04_simple_Formation/Data Bus /For matrix Plot10 ==
  T : Inport
  MATLAB Function : MATLAB Function  TreatAsAtomicUnit=on
  To Workspace : ToWorkspace  VariableName=T3  SaveFormat=Structure With Time  SampleTime=-1
  wires:
  T/1 -> MATLAB Function/1(u)
  MATLAB Function/1(y) -> To Workspace/1

== system CAMFC2_04_simple_Formation/Data Bus /For matrix Plot11 ==
  T : Inport
  MATLAB Function : MATLAB Function  TreatAsAtomicUnit=on
  To Workspace : ToWorkspace  VariableName=T4  SaveFormat=Structure With Time  SampleTime=-1
  wires:
  MATLAB Function/1(y) -> To Workspace/1
  T/1 -> MATLAB Function/1(u)

== system CAMFC2_04_simple_Formation/Data Bus /For matrix Plot12 ==
  epsilon : Inport
  MATLAB Function : MATLAB Function  TreatAsAtomicUnit=on
  To Workspace : ToWorkspace  VariableName=epsilon1  SaveFormat=Structure With Time  SampleTime=-1
  wires:
  epsilon/1 -> MATLAB Function/1(u)
  MATLAB Function/1(y) -> To Workspace/1

== system CAMFC2_04_simple_Formation/Data Bus /For matrix Plot13 ==
  epsilon : Inport
  MATLAB Function : MATLAB Function  TreatAsAtomicUnit=on
  To Workspace : ToWorkspace  VariableName=epsilon2  SaveFormat=Structure With Time  SampleTime=-1
  wires:
  MATLAB Function/1(y) -> To Workspace/1
  epsilon/1 -> MATLAB Function/1(u)

== system CAMFC2_04_simple_Formation/Data Bus /For matrix Plot14 ==
  epsilon : Inport
  MATLAB Function : MATLAB Function  TreatAsAtomicUnit=on
  To Workspace : ToWorkspace  VariableName=epsilon3  SaveFormat=Structure With Time  SampleTime=-1
  wires:
  MATLAB Function/1(y) -> To Workspace/1
  epsilon/1 -> MATLAB Function/1(u)

== system CAMFC2_04_simple_Formation/Data Bus /For matrix Plot15 ==
  epsilon : Inport
  MATLAB Function : MATLAB Function  TreatAsAtomicUnit=on
  To Workspace : ToWorkspace  VariableName=epsilon4  SaveFormat=Structure With Time  SampleTime=-1
  wires:
  epsilon/1 -> MATLAB Function/1(u)
  MATLAB Function/1(y) -> To Workspace/1

== system CAMFC2_04_simple_Formation/Data Bus /For matrix Plot16 ==
  epsilon : Inport
  MATLAB Function : MATLAB Function  TreatAsAtomicUnit=on
  To Workspace : ToWorkspace  VariableName=epsilon5  SaveFormat=Structure With Time  SampleTime=-1
  wires:
  epsilon/1 -> MATLAB Function/1(u)
  MATLAB Function/1(y) -> To Workspace/1

== system CAMFC2_04_simple_Formation/Data Bus /For matrix Plot17 ==
  epsilon : Inport
  MATLAB Function : MATLAB Function  TreatAsAtomicUnit=on
  To Workspace : ToWorkspace  VariableName=epsilon6  SaveFormat=Structure With Time  SampleTime=-1
  wires:
  MATLAB Function/1(y) -> To Workspace/1
  epsilon/1 -> MATLAB Function/1(u)

== system CAMFC2_04_simple_Formation/Data Bus /For matrix Plot18 ==
  P : Inport
  MATLAB Function : MATLAB Function  TreatAsAtomicUnit=on
  Scope17 : Scope
  To Workspace : ToWorkspace  VariableName=P5  SaveFormat=Structure With Time  SampleTime=-1
  wires:
  MATLAB Function/1(y) -> To Workspace/1, Scope17/1
  P/1 -> MATLAB Function/1(u)

== system CAMFC2_04_simple_Formation/Data Bus /For matrix Plot19 ==
  P : Inport
  MATLAB Function : MATLAB Function  TreatAsAtomicUnit=on
  To Workspace : ToWorkspace  VariableName=P6  SaveFormat=Structure With Time  SampleTime=-1
  wires:
  P/1 -> MATLAB Function/1(u)
  MATLAB Function/1(y) -> To Workspace/1

== system CAMFC2_04_simple_Formation/Data Bus /For matrix Plot2 ==
  P : Inport
  MATLAB Function : MATLAB Function  TreatAsAtomicUnit=on
  To Workspace : ToWorkspace  VariableName=P3  SaveFormat=Structure With Time  SampleTime=-1
  wires:
  MATLAB Function/1(y) -> To Workspace/1
  P/1 -> MATLAB Function/1(u)

== system CAMFC2_04_simple_Formation/Data Bus /For matrix Plot20 ==
  T : Inport
  MATLAB Function : MATLAB Function  TreatAsAtomicUnit=on
  To Workspace : ToWorkspace  VariableName=T5  SaveFormat=Structure With Time  SampleTime=-1
  wires:
  MATLAB Function/1(y) -> To Workspace/1
  T/1 -> MATLAB Function/1(u)

== system CAMFC2_04_simple_Formation/Data Bus /For matrix Plot21 ==
  T : Inport
  MATLAB Function : MATLAB Function  TreatAsAtomicUnit=on
  To Workspace : ToWorkspace  VariableName=T6  SaveFormat=Structure With Time  SampleTime=-1
  wires:
  T/1 -> MATLAB Function/1(u)
  MATLAB Function/1(y) -> To Workspace/1

== system CAMFC2_04_simple_Formation/Data Bus /For matrix Plot22 ==
  A_hat : Inport
  MATLAB Function : MATLAB Function  TreatAsAtomicUnit=on
  Scope17 : Scope
  To Workspace : ToWorkspace  VariableName=A_hat5  SaveFormat=Structure With Time  SampleTime=-1
  wires:
  MATLAB Function/1(y) -> To Workspace/1, Scope17/1
  A_hat/1 -> MATLAB Function/1(u)

== system CAMFC2_04_simple_Formation/Data Bus /For matrix Plot23 ==
  A_hat : Inport
  MATLAB Function : MATLAB Function  TreatAsAtomicUnit=on
  Scope17 : Scope
  To Workspace : ToWorkspace  VariableName=A_hat6  SaveFormat=Structure With Time  SampleTime=-1
  wires:
  A_hat/1 -> MATLAB Function/1(u)
  MATLAB Function/1(y) -> Scope17/1, To Workspace/1

== system CAMFC2_04_simple_Formation/Data Bus /For matrix Plot3 ==
  P : Inport
  MATLAB Function : MATLAB Function  TreatAsAtomicUnit=on
  Scope17 : Scope
  To Workspace : ToWorkspace  VariableName=P4  SaveFormat=Structure With Time  SampleTime=-1
  wires:
  P/1 -> MATLAB Function/1(u)
  MATLAB Function/1(y) -> Scope17/1, To Workspace/1

== system CAMFC2_04_simple_Formation/Data Bus /For matrix Plot4 ==
  A_hat : Inport
  MATLAB Function : MATLAB Function  TreatAsAtomicUnit=on
  Scope17 : Scope
  To Workspace : ToWorkspace  VariableName=A_hat1  SaveFormat=Structure With Time  SampleTime=-1
  wires:
  MATLAB Function/1(y) -> Scope17/1, To Workspace/1
  A_hat/1 -> MATLAB Function/1(u)

== system CAMFC2_04_simple_Formation/Data Bus /For matrix Plot5 ==
  A_hat : Inport
  MATLAB Function : MATLAB Function  TreatAsAtomicUnit=on
  To Workspace : ToWorkspace  VariableName=A_hat2  SaveFormat=Structure With Time  SampleTime=-1
  wires:
  A_hat/1 -> MATLAB Function/1(u)
  MATLAB Function/1(y) -> To Workspace/1

== system CAMFC2_04_simple_Formation/Data Bus /For matrix Plot6 ==
  A_hat : Inport
  MATLAB Function : MATLAB Function  TreatAsAtomicUnit=on
  To Workspace : ToWorkspace  VariableName=A_hat3  SaveFormat=Structure With Time  SampleTime=-1
  wires:
  MATLAB Function/1(y) -> To Workspace/1
  A_hat/1 -> MATLAB Function/1(u)

== system CAMFC2_04_simple_Formation/Data Bus /For matrix Plot7 ==
  A_hat : Inport
  MATLAB Function : MATLAB Function  TreatAsAtomicUnit=on
  Scope17 : Scope
  To Workspace : ToWorkspace  VariableName=A_hat4  SaveFormat=Structure With Time  SampleTime=-1
  wires:
  A_hat/1 -> MATLAB Function/1(u)
  MATLAB Function/1(y) -> Scope17/1, To Workspace/1

== system CAMFC2_04_simple_Formation/Data Bus /For matrix Plot8 ==
  T : Inport
  MATLAB Function : MATLAB Function  TreatAsAtomicUnit=on
  Scope17 : Scope
  To Workspace : ToWorkspace  VariableName=T1  SaveFormat=Structure With Time  SampleTime=-1
  wires:
  MATLAB Function/1(y) -> Scope17/1, To Workspace/1
  T/1 -> MATLAB Function/1(u)

== system CAMFC2_04_simple_Formation/Data Bus /For matrix Plot9 ==
  T : Inport
  MATLAB Function : MATLAB Function  TreatAsAtomicUnit=on
  To Workspace : ToWorkspace  VariableName=T2  SaveFormat=Structure With Time  SampleTime=-1
  wires:
  T/1 -> MATLAB Function/1(u)
  MATLAB Function/1(y) -> To Workspace/1

== system CAMFC2_04_simple_Formation/Data Bus /Reference Trajectory ==
  Constant2 : Constant  Value=2
  Constant5 : Constant
  Mux : Mux  Inputs=2
  Pulse Generator : DiscretePulseGenerator  PulseType=Time based  Amplitude=2  Period=20  PulseWidth=50
  X1 : Sin  Amplitude=3  Frequency=0.5  SampleTime=0
  X0 : Outport
  wires:
  ? -> Mux/1
  Mux/1 -> X0/1
  ? -> Mux/2

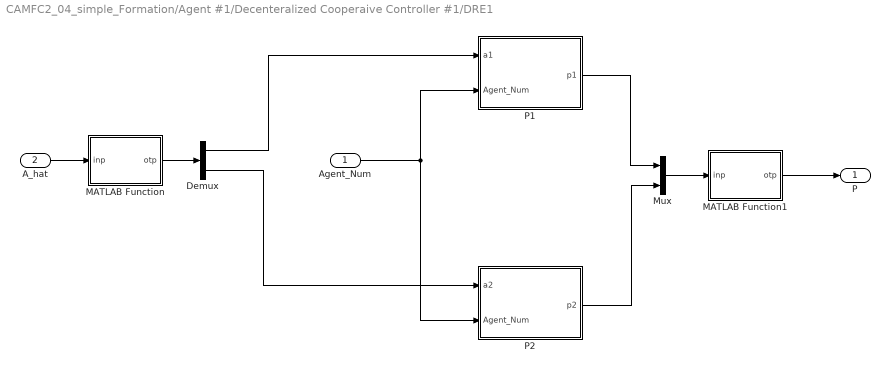
== system CAMFC2_04_simple_Formation/Agent #1/Decenteralized Cooperaive Controller #1/DRE1 ==
  Agent_Num : Inport
  A_hat : Inport  Port=2
  Demux : Demux  Outputs=n
  MATLAB Function : MATLAB Function  TreatAsAtomicUnit=on
  MATLAB Function1 : MATLAB Function  TreatAsAtomicUnit=on
  Mux : Mux  Inputs=2
  P1 : Subsystem
  P2 : Subsystem
  P : Outport
  wires:
  Demux/1 -> P1/1(a1)
  Demux/2 -> P2/1(a2)
  P2/1(p2) -> Mux/2
  Agent_Num/1 -> P1/2(Agent_Num), P2/2(Agent_Num)
  A_hat/1 -> MATLAB Function/1(inp)
  MATLAB Function/1(otp) -> Demux/1
  P1/1(p1) -> Mux/1
  Mux/1 -> MATLAB Function1/1(inp)
  MATLAB Function1/1(otp) -> P/1

== system CAMFC2_04_simple_Formation/Agent #1/Decenteralized Cooperaive Controller #1/Differentiator1 ==
  x_d : Inport
  Integrator : Integrator  InitialCondition=zeros(n0,1)
  Integrator1 : Integrator  InitialCondition=zeros(n0,1)
  Sliding differentiator : MATLAB Function  TreatAsAtomicUnit=on
  Sliding differentiator1 : MATLAB Function  TreatAsAtomicUnit=on
  Sum : Sum  Inputs=|-+
  Dx_d : Outport
  wires:
  Sliding differentiator/1(u) -> Integrator1/1, Dx_d/1
  Sliding differentiator1/1(Du1) -> Integrator/1
  Integrator/1 -> Sliding differentiator/1(u1)
  x_d/1 -> Sum/1
  Sum/1 -> Sliding differentiator/2(e), Sliding differentiator1/1(e)
  Integrator1/1 -> Sum/2

== system CAMFC2_04_simple_Formation/Agent #1/Decenteralized Cooperaive Controller #1/Differentiator2 ==
  x_d : Inport
  Integrator : Integrator  InitialCondition=zeros(N+1,n)
  Integrator1 : Integrator  InitialCondition=zeros(N+1,n)
  Sliding differentiator : MATLAB Function  TreatAsAtomicUnit=on
  Sliding differentiator1 : MATLAB Function  TreatAsAtomicUnit=on
  Sum : Sum  Inputs=|-+
  Dx_d : Outport
  wires:
  Sliding differentiator/1(u) -> Integrator1/1, Dx_d/1
  Sliding differentiator1/1(Du1) -> Integrator/1
  Integrator/1 -> Sliding differentiator/1(u1)
  x_d/1 -> Sum/1
  Sum/1 -> Sliding differentiator/2(e), Sliding differentiator1/1(e)
  Integrator1/1 -> Sum/2

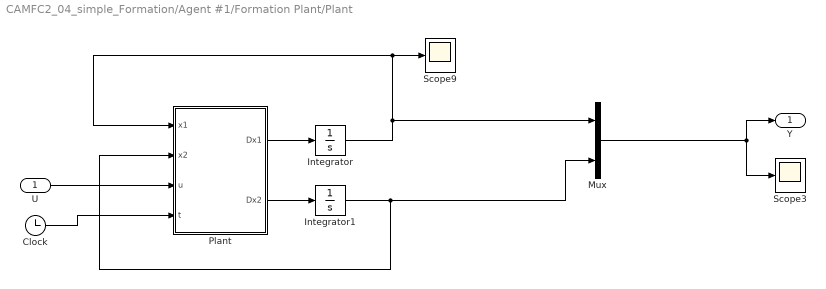
== system CAMFC2_04_simple_Formation/Agent #1/Formation Plant/Plant ==
  U : Inport
  Clock : Clock
  Integrator : Integrator  InitialCondition=6
  Integrator1 : Integrator  InitialCondition=2
  Mux : Mux  Inputs=2
  Plant : MATLAB Function  TreatAsAtomicUnit=on
  Scope3 : Scope
  Scope9 : Scope
  Y : Outport
  wires:
  Plant/1(Dx1) -> Integrator/1
  U/1 -> Plant/3(u)
  Plant/2(Dx2) -> Integrator1/1
  Clock/1 -> Plant/4(t)
  Integrator/1 -> Mux/1, Plant/1(x1), Scope9/1
  Integrator1/1 -> Mux/2, Plant/2(x2)
  Mux/1 -> Y/1, Scope3/1

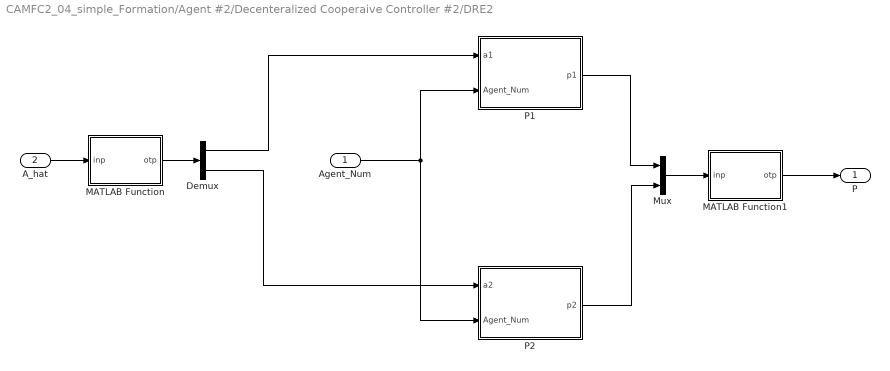
== system CAMFC2_04_simple_Formation/Agent #2/Decenteralized Cooperaive Controller #2/DRE2 ==
  Agent_Num : Inport
  A_hat : Inport  Port=2
  Demux : Demux  Outputs=n
  MATLAB Function : MATLAB Function  TreatAsAtomicUnit=on
  MATLAB Function1 : MATLAB Function  TreatAsAtomicUnit=on
  Mux : Mux  Inputs=2
  P1 : Subsystem
  P2 : Subsystem
  P : Outport
  wires:
  Demux/1 -> P1/1(a1)
  Demux/2 -> P2/1(a2)
  P2/1(p2) -> Mux/2
  Agent_Num/1 -> P1/2(Agent_Num), P2/2(Agent_Num)
  A_hat/1 -> MATLAB Function/1(inp)
  MATLAB Function/1(otp) -> Demux/1
  P1/1(p1) -> Mux/1
  Mux/1 -> MATLAB Function1/1(inp)
  MATLAB Function1/1(otp) -> P/1

== system CAMFC2_04_simple_Formation/Agent #2/Decenteralized Cooperaive Controller #2/Differentiator1 ==
  x_d : Inport
  Integrator : Integrator  InitialCondition=zeros(n0,1)
  Integrator1 : Integrator  InitialCondition=zeros(n0,1)
  Sliding differentiator : MATLAB Function  TreatAsAtomicUnit=on
  Sliding differentiator1 : MATLAB Function  TreatAsAtomicUnit=on
  Sum : Sum  Inputs=|-+
  Dx_d : Outport
  wires:
  Sliding differentiator/1(u) -> Integrator1/1, Dx_d/1
  Sliding differentiator1/1(Du1) -> Integrator/1
  Integrator/1 -> Sliding differentiator/1(u1)
  x_d/1 -> Sum/1
  Sum/1 -> Sliding differentiator/2(e), Sliding differentiator1/1(e)
  Integrator1/1 -> Sum/2

== system CAMFC2_04_simple_Formation/Agent #2/Decenteralized Cooperaive Controller #2/Differentiator2 ==
  x_d : Inport
  Integrator : Integrator  InitialCondition=zeros(N+1,n)
  Integrator1 : Integrator  InitialCondition=zeros(N+1,n)
  Sliding differentiator : MATLAB Function  TreatAsAtomicUnit=on
  Sliding differentiator1 : MATLAB Function  TreatAsAtomicUnit=on
  Sum : Sum  Inputs=|-+
  Dx_d : Outport
  wires:
  Sliding differentiator/1(u) -> Integrator1/1, Dx_d/1
  Sliding differentiator1/1(Du1) -> Integrator/1
  Integrator/1 -> Sliding differentiator/1(u1)
  x_d/1 -> Sum/1
  Sum/1 -> Sliding differentiator/2(e), Sliding differentiator1/1(e)
  Integrator1/1 -> Sum/2

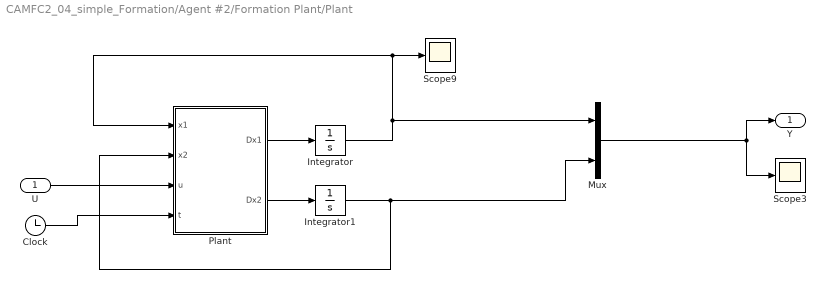
== system CAMFC2_04_simple_Formation/Agent #2/Formation Plant/Plant ==
  U : Inport
  Clock : Clock
  Integrator : Integrator  InitialCondition=3
  Integrator1 : Integrator  InitialCondition=3*sqrt(3)
  Mux : Mux  Inputs=2
  Plant : MATLAB Function  TreatAsAtomicUnit=on
  Scope3 : Scope
  Scope9 : Scope
  Y : Outport
  wires:
  Plant/1(Dx1) -> Integrator/1
  U/1 -> Plant/3(u)
  Plant/2(Dx2) -> Integrator1/1
  Clock/1 -> Plant/4(t)
  Integrator/1 -> Mux/1, Plant/1(x1), Scope9/1
  Integrator1/1 -> Mux/2, Plant/2(x2)
  Mux/1 -> Y/1, Scope3/1

== system CAMFC2_04_simple_Formation/Agent #3/Decenteralized Cooperaive Controller #3/DRE3 ==
  Agent_Num : Inport
  A_hat : Inport  Port=2
  Demux : Demux  Outputs=n
  MATLAB Function : MATLAB Function  TreatAsAtomicUnit=on
  MATLAB Function1 : MATLAB Function  TreatAsAtomicUnit=on
  Mux : Mux  Inputs=2
  P1 : Subsystem
  P2 : Subsystem
  P : Outport
  wires:
  Demux/1 -> P1/1(a1)
  Demux/2 -> P2/1(a2)
  P2/1(p2) -> Mux/2
  Agent_Num/1 -> P1/2(Agent_Num), P2/2(Agent_Num)
  A_hat/1 -> MATLAB Function/1(inp)
  MATLAB Function/1(otp) -> Demux/1
  P1/1(p1) -> Mux/1
  Mux/1 -> MATLAB Function1/1(inp)
  MATLAB Function1/1(otp) -> P/1

== system CAMFC2_04_simple_Formation/Agent #3/Decenteralized Cooperaive Controller #3/Differentiator2 ==
  x_d : Inport
  Integrator : Integrator  InitialCondition=zeros(N+1,n)
  Integrator1 : Integrator  InitialCondition=zeros(N+1,n)
  Sliding differentiator : MATLAB Function  TreatAsAtomicUnit=on
  Sliding differentiator1 : MATLAB Function  TreatAsAtomicUnit=on
  Sum : Sum  Inputs=|-+
  Dx_d : Outport
  wires:
  Sliding differentiator/1(u) -> Integrator1/1, Dx_d/1
  Sliding differentiator1/1(Du1) -> Integrator/1
  Integrator/1 -> Sliding differentiator/1(u1)
  x_d/1 -> Sum/1
  Sum/1 -> Sliding differentiator/2(e), Sliding differentiator1/1(e)
  Integrator1/1 -> Sum/2

== system CAMFC2_04_simple_Formation/Agent #3/Decenteralized Cooperaive Controller #3/Differentiator3 ==
  x_d : Inport
  Integrator : Integrator  InitialCondition=zeros(n0,1)
  Integrator1 : Integrator  InitialCondition=zeros(n0,1)
  Sliding differentiator : MATLAB Function  TreatAsAtomicUnit=on
  Sliding differentiator1 : MATLAB Function  TreatAsAtomicUnit=on
  Sum : Sum  Inputs=|-+
  Dx_d : Outport
  wires:
  Sliding differentiator/1(u) -> Integrator1/1, Dx_d/1
  Sliding differentiator1/1(Du1) -> Integrator/1
  Integrator/1 -> Sliding differentiator/1(u1)
  x_d/1 -> Sum/1
  Sum/1 -> Sliding differentiator/2(e), Sliding differentiator1/1(e)
  Integrator1/1 -> Sum/2

== system CAMFC2_04_simple_Formation/Agent #3/Formation Plant/Plant ==
  U : Inport
  Clock : Clock
  Integrator : Integrator  InitialCondition=-3
  Integrator1 : Integrator  InitialCondition=3*sqrt(3)
  Mux : Mux  Inputs=2
  Plant : MATLAB Function  TreatAsAtomicUnit=on
  Scope3 : Scope
  Scope9 : Scope
  Y : Outport
  wires:
  Plant/1(Dx1) -> Integrator/1
  U/1 -> Plant/3(u)
  Plant/2(Dx2) -> Integrator1/1
  Clock/1 -> Plant/4(t)
  Integrator/1 -> Mux/1, Plant/1(x1), Scope9/1
  Integrator1/1 -> Mux/2, Plant/2(x2)
  Mux/1 -> Y/1, Scope3/1

== system CAMFC2_04_simple_Formation/Agent #4/Decenteralized Cooperaive Controller #4/DRE4 ==
  Agent_Num : Inport
  A_hat : Inport  Port=2
  Demux : Demux  Outputs=n
  MATLAB Function : MATLAB Function  TreatAsAtomicUnit=on
  MATLAB Function1 : MATLAB Function  TreatAsAtomicUnit=on
  Mux : Mux  Inputs=2
  P1 : Subsystem
  P2 : Subsystem
  P : Outport
  wires:
  Demux/1 -> P1/1(a1)
  Demux/2 -> P2/1(a2)
  P2/1(p2) -> Mux/2
  Agent_Num/1 -> P1/2(Agent_Num), P2/2(Agent_Num)
  A_hat/1 -> MATLAB Function/1(inp)
  MATLAB Function/1(otp) -> Demux/1
  P1/1(p1) -> Mux/1
  Mux/1 -> MATLAB Function1/1(inp)
  MATLAB Function1/1(otp) -> P/1

== system CAMFC2_04_simple_Formation/Agent #4/Decenteralized Cooperaive Controller #4/Differentiator0 ==
  x_d : Inport
  Integrator : Integrator
  Integrator1 : Integrator
  Sliding differentiator : MATLAB Function  TreatAsAtomicUnit=on
  Sliding differentiator1 : MATLAB Function  TreatAsAtomicUnit=on
  Sum : Sum  Inputs=|-+
  Dx_d : Outport
  wires:
  Sliding differentiator/1(u) -> Integrator1/1, Dx_d/1
  Sliding differentiator1/1(Du1) -> Integrator/1
  Integrator/1 -> Sliding differentiator/1(u1)
  x_d/1 -> Sum/1
  Sum/1 -> Sliding differentiator/2(e), Sliding differentiator1/1(e)
  Integrator1/1 -> Sum/2
